simulink model "dc_motor"  (R2017a)
settings: Solver=ode45  StartTime=0.0  StopTime=3  RelTol=1e-3
undefined symbols (not defined in the file): b, J, K, L, R
settings Model: Creator=sansh  LastModifiedBy=sansh

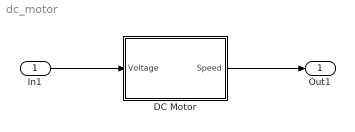
== system dc_motor ==
  In1 : Inport
  DC Motor : Subsystem
  Out1 : Outport
  wires:
  In1/1 -> DC Motor/1(Voltage)
  DC Motor/1(Speed) -> Out1/1

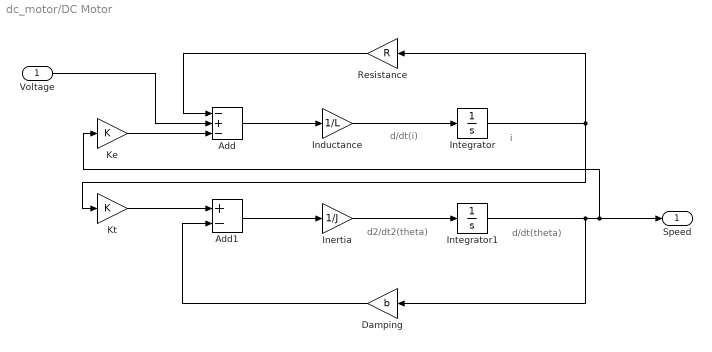
== system dc_motor/DC Motor ==
  note: i
  note: d/dt(i)
  note: d/dt(theta)
  note: d2/dt2(theta)
  Voltage : Inport
  Add : Sum  Inputs=-+-
  Add1 : Sum  Inputs=+-
  Damping : Gain  Gain=b
  Inductance : Gain  Gain=1/L
  Inertia : Gain  Gain=1/J
  Integrator : Integrator
  Integrator1 : Integrator
  Ke : Gain  Gain=K
  Kt : Gain  Gain=K
  Resistance : Gain  Gain=R
  Speed : Outport
  wires:
  Inductance/1 -> Integrator/1
  Integrator1/1 -> Damping/1, Speed/1, Ke/1
  Inertia/1 -> Integrator1/1
  Integrator/1 -> Resistance/1, Kt/1
  Kt/1 -> Add1/1
  Voltage/1 -> Add/2
  Resistance/1 -> Add/1
  Damping/1 -> Add1/2
  Ke/1 -> Add/3
  Add/1 -> Inductance/1
  Add1/1 -> Inertia/1
